simulink model "ccSim"  (R2015a)
settings: Solver=ode45  StartTime=0.0  StopTime=100  MaxStep=0.001  RelTol=1e-3
values from neighbouring files (symbols this model uses):
  D = 3.0/100    (= 0.03)    [initfile.m]
undefined symbols (not defined in the file or in its folder): M_inv, nu_0
settings Model: CovModelRefEnable=off  Creator=risendal  LastModifiedBy=risendal
settings DataIOCC: SaveFormat=Dataset
settings HardwareCC: ProdBitPerPointer=64  ProdLargestAtomicFloat=Float  ProdIntDivRoundTo=Zero  ProdEndianess=LittleEndian  ProdHWDeviceType=Specified
settings GRTTargetCC: GeneratePreprocessorConditionals=Use local settings

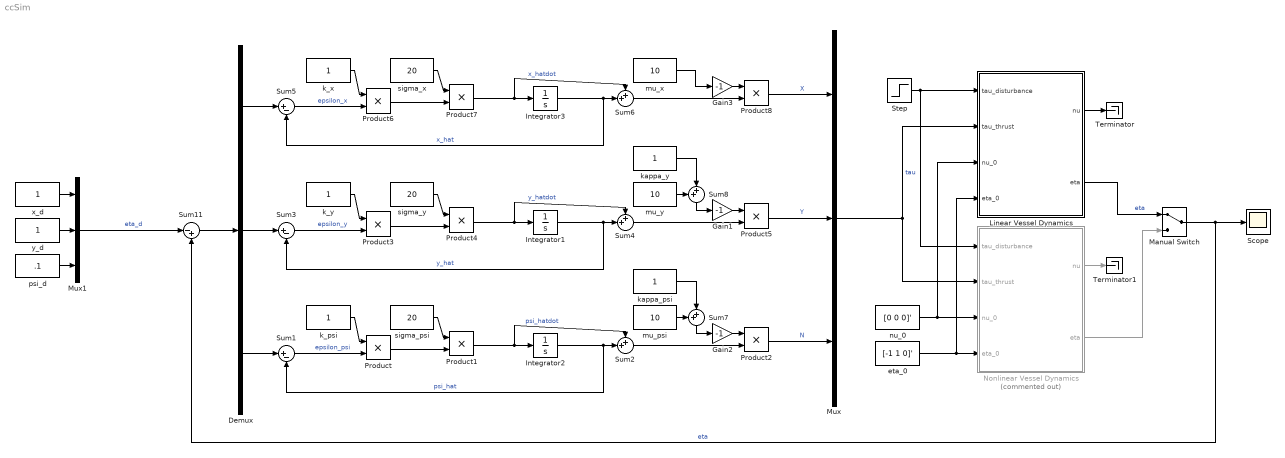
== system ccSim ==
  Demux : Demux  Outputs=3
  Gain1 : Gain  Gain=-1
  Gain2 : Gain  Gain=-1
  Gain3 : Gain  Gain=-1
  Integrator1 : Integrator
  Integrator2 : Integrator
  Integrator3 : Integrator
  "Linear Vessel Dynamics " : Subsystem
  Manual Switch : ManualSwitch
  Mux : Mux  Inputs=3
  Mux1 : Mux  Inputs=3
  Nonlinear Vessel Dynamics : Subsystem  Commented=on
  Product{,1..8} (9 alike) : Product
  Scope : Scope
      settings: TimeRange=auto  MaxDataPoints=5000  SaveToWorkspace=off  SaveName=ScopeData  YMin=0  YMax=3.5  SampleTime=-1
  Step : Step  Time=60  Before=[0 0 0]'  After=[.3 .3 0]'  SampleTime=0
  Sum1 : Sum  Inputs=|+-
  Sum11 : Sum  Inputs=|-+
  Sum{2,4,6..8} (5 alike) : Sum  Inputs=++|
  Sum3 : Sum  Inputs=|+-
  Sum5 : Sum  Inputs=|+-
  Terminator : Terminator
  Terminator1 : Terminator
  eta_0 : Constant  Value=[-1 1 0]'
  k_psi : Constant
  k_x : Constant
  k_y : Constant
  kappa_psi : Constant
  kappa_y : Constant
  mu_psi : Constant  Value=10
  mu_x : Constant  Value=10
  mu_y : Constant  Value=10
  nu_0 : Constant  Value=[0 0 0]'
  psi_d : Constant  Value=.1
  sigma_psi : Constant  Value=20
  sigma_x : Constant  Value=20
  sigma_y : Constant  Value=20
  x_d : Constant
  y_d : Constant
  wires:
  Integrator2/1 -> Sum1/2, Sum2/2  "psi_hat"
  Product1/1 -> Integrator2/1, Sum2/1  "psi_hatdot"
  Product/1 -> Product1/2
  Sum1/1 -> Product/2  "epsilon_psi"
  Sum2/1 -> Product2/2
  psi_d/1 -> Mux1/3
  Sum11/1 -> Demux/1
  Manual Switch/1 -> Scope/1, Sum11/2  "eta"
  Step/1 -> "Linear Vessel Dynamics "/1(tau_disturbance), Nonlinear Vessel Dynamics/1(tau_disturbance)
  Mux/1 -> "Linear Vessel Dynamics "/2(tau_thrust), Nonlinear Vessel Dynamics/2(tau_thrust)  "tau"
  Product2/1 -> Mux/3  "N"
  Demux/3 -> Sum1/1
  y_d/1 -> Mux1/2
  x_d/1 -> Mux1/1
  Mux1/1 -> Sum11/1  "eta_d"
  k_psi/1 -> Product/1
  sigma_psi/1 -> Product1/1
  Gain2/1 -> Product2/1
  Sum7/1 -> Gain2/1
  mu_psi/1 -> Sum7/1
  kappa_psi/1 -> Sum7/2
  Integrator1/1 -> Sum3/2, Sum4/2  "y_hat"
  Product4/1 -> Integrator1/1, Sum4/1  "y_hatdot"
  Product3/1 -> Product4/2
  Sum3/1 -> Product3/2  "epsilon_y"
  Sum4/1 -> Product5/2
  Demux/2 -> Sum3/1
  k_y/1 -> Product3/1
  sigma_y/1 -> Product4/1
  Gain1/1 -> Product5/1
  Sum8/1 -> Gain1/1
  mu_y/1 -> Sum8/1
  kappa_y/1 -> Sum8/2
  Product5/1 -> Mux/2  "Y"
  Integrator3/1 -> Sum5/2, Sum6/2  "x_hat"
  Product7/1 -> Integrator3/1, Sum6/1  "x_hatdot"
  Product6/1 -> Product7/2
  Sum5/1 -> Product6/2  "epsilon_x"
  Sum6/1 -> Product8/2
  Demux/1 -> Sum5/1
  k_x/1 -> Product6/1
  sigma_x/1 -> Product7/1
  Gain3/1 -> Product8/1
  mu_x/1 -> Gain3/1
  Product8/1 -> Mux/1  "X"
  "Linear Vessel Dynamics "/1(nu) -> Terminator/1
  Nonlinear Vessel Dynamics/1(nu) -> Terminator1/1
  Nonlinear Vessel Dynamics/2(eta) -> Manual Switch/2
  "Linear Vessel Dynamics "/2(eta) -> Manual Switch/1  "eta"
  nu_0/1 -> "Linear Vessel Dynamics "/3(nu_0), Nonlinear Vessel Dynamics/3(nu_0)
  eta_0/1 -> "Linear Vessel Dynamics "/4("eta_0 "), Nonlinear Vessel Dynamics/4("eta_0 ")

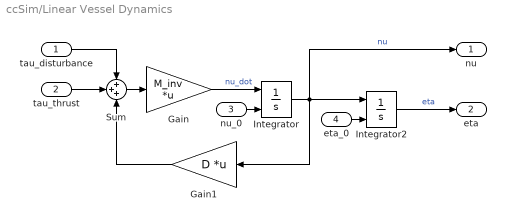
== system ccSim/Linear Vessel Dynamics  ==
  tau_disturbance : Inport
  tau_thrust : Inport  Port=2
  nu_0 : Inport  Port=3
  "eta_0 " : Inport  Port=4
  Gain : Gain  Gain=M_inv  Multiplication=Matrix(K*u)
  Gain1 : Gain  Gain=D  Multiplication=Matrix(K*u)
  Integrator : Integrator  InitialConditionSource=external  InitialCondition=nu_0
  Integrator2 : Integrator  InitialConditionSource=external  InitialCondition=nu_0
  Sum : Sum  Inputs=+++
  nu : Outport
  eta : Outport  Port=2
  wires:
  Integrator/1 -> Integrator2/1, nu/1, Gain1/1  "nu"
  Gain/1 -> Integrator/1  "nu_dot"
  Sum/1 -> Gain/1
  Gain1/1 -> Sum/3
  tau_thrust/1 -> Sum/2
  Integrator2/1 -> eta/1  "eta"
  tau_disturbance/1 -> Sum/1
  nu_0/1 -> Integrator/2
  "eta_0 "/1 -> Integrator2/2

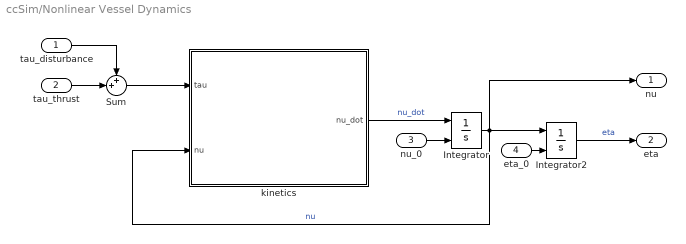
== system ccSim/Nonlinear Vessel Dynamics ==
  tau_disturbance : Inport
  tau_thrust : Inport  Port=2
  nu_0 : Inport  Port=3
  "eta_0 " : Inport  Port=4
  Integrator : Integrator  InitialConditionSource=external  InitialCondition=nu_0
  Integrator2 : Integrator  InitialConditionSource=external  InitialCondition=nu_0
  Sum : Sum  Inputs=++|
  kinetics : MATLAB Function  TreatAsAtomicUnit=on
      settings: PermitHierarchicalResolution=ParametersOnly
  nu : Outport
  eta : Outport  Port=2
  wires:
  Integrator/1 -> kinetics/2(nu), Integrator2/1, nu/1  "nu"
  kinetics/1(nu_dot) -> Integrator/1  "nu_dot"
  Sum/1 -> kinetics/1(tau)
  tau_thrust/1 -> Sum/2
  Integrator2/1 -> eta/1  "eta"
  tau_disturbance/1 -> Sum/1
  nu_0/1 -> Integrator/2
  "eta_0 "/1 -> Integrator2/2

== matlab function ccSim/Nonlinear Vessel Dynamics/kinetics ==
  data: tau input; nu_dot output; nu input
function nu_dot = CSAD_nu_dot(tau,nu)

u   = nu(1);
v   = nu(2);
r   = nu(3);


%% MATRICES

m    = 127.92;   I_z  = 61.967;   x_g = 0; %0.0432;


%% Added mass
X_ud  =   3.262;											
					Y_vd =      28.89;	N_vd =    0.157;		
					Y_rd =      0.525;	N_rd =    13.98;

%% Total mass matrix
m_11 = m-X_ud;
m_22 = m-Y_vd;
m_23 = m*x_g-Y_rd;
m_32 = m*x_g-N_vd;
m_33 = I_z-N_rd;

M    = [m_11 0    0
        0    m_22 m_23
        0    m_32 m_33]
	
%% DAMPING 

% Surge:
% Based on fitting of towing data from -0.8 < u < 0.8 m/s
X_u     = -2.332;
X_uu	=  0;
X_uuu	= -8.557;

% Sway:
% Based on fitting of towing data from -0.45 < u < 0.45 m/s
Y_v 	= -4.673;
Y_vv	=  0.3976;
Y_vvv	= -313.3;

% Yaw:
% Based on fitting of towing data from -8 < u < 8 deg/s
% The fitting range is limited. Towing should be performed for higher
% velocities.
N_r		= -0.01675;
N_rr	= -0.01148;
N_rrr	= -0.0003578;

% Y_vvv og N_rrr er fra curvefitting uten minus, men ser ut til å fungere
% med minus. 
                           N_v		= 0;                Y_r	    =  -7.250; 
                           N_vv	    = -0.2088;          Y_rr	=  -3.450;
                           N_vvv	= 0;                Y_rrr	=  0;
						
						   Y_rv	    = -0.805;			Y_vr	=  -0.845; 

						   N_rv	    = 0.08;             N_vr	= 0.08;
                           

%% Correolis matrix
c_13 = -(m-Y_vd)*v-(m*x_g-Y_rd)*r;
c_23 = (m-X_ud)*u;

C    = [0     0     c_13
        0     0     c_23
        -c_13 -c_23 0   ];

%% Assembly of the damping matrix
d_11 = X_u + X_uu*abs(u) + X_uuu*u^2;
d_22 = Y_v + Y_vv*abs(v) + Y_vvv*v^2;
d_33 = N_r + N_rr*abs(r) + N_rrr*r^2;

d_23 = 0; % Y_r + Y_rr*abs(r) + Y_rrr*r^2 + Y_vr*abs(v); Not verified, temporarily disabled
d_32 = 0; % N_v + N_vv*abs(v) + N_vvv*v^2 + N_rv*abs(r); Not verified, temporarily disabled

D    = - [d_11 0    0
          0    d_22 d_23
          0    d_32 d_33]

%% CALCULATION
nu_dot = M\(tau-D*nu);
